simulink model "ILC_pend"  (R2018a)
settings: Solver=ode1  StartTime=0.0  StopTime=10.0  FixedStep=.002  RelTol=1e-3
undefined symbols (not defined in the file or in its folder): A, B, C, D, K
settings Model: Creator=capn  LastModifiedBy=barre
settings CodeAppCC: StateflowObjectComments=on

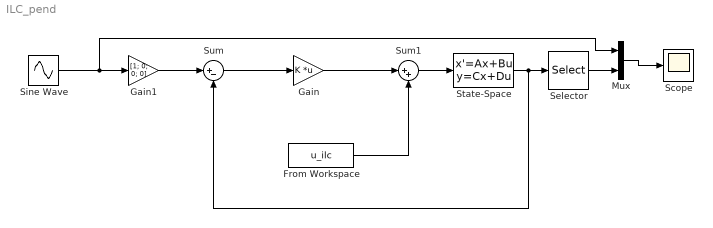
== system ILC_pend ==
  From Workspace : FromWorkspace  VariableName=u_ilc  SampleTime=0
  Gain : Gain  Gain=K  Multiplication=Matrix(K*u)
  Gain1 : Gain  Gain=[1; 0; 0; 0]
  Mux : Mux  Inputs=2
  Scope : Scope
  Selector : Selector  InputPortWidth=4  IndexOptions=Index vector (dialog)  Indices=[1 ]  OutputSizes=1
  Sine Wave : Sin  SampleTime=0
  State-Space : StateSpace  A=A  B=B  C=C  D=D  InitialCondition=[ 0 0 0 0]
  Sum : Sum  Inputs=|+-
  Sum1 : Sum  Inputs=|++
  wires:
  Gain/1 -> Sum1/1
  Sum1/1 -> State-Space/1
  Sine Wave/1 -> Mux/1, Gain1/1
  Mux/1 -> Scope/1
  Sum/1 -> Gain/1
  Gain1/1 -> Sum/1
  State-Space/1 -> Sum/2, Selector/1
  Selector/1 -> Mux/2
  From Workspace/1 -> Sum1/2
